simulink subsystem "ProcNav"  (R2020a)
settings: Solver=VariableStepAuto  StartTime=0.0  StopTime=10.0  RelTol=1e-3
undefined symbols (not defined in the file): DiscIntNeverNeededParam
libraries: aerolibutil x3, sharedtransform x2
settings Model: Creator=Lamarre  LastModifiedBy=lamarre

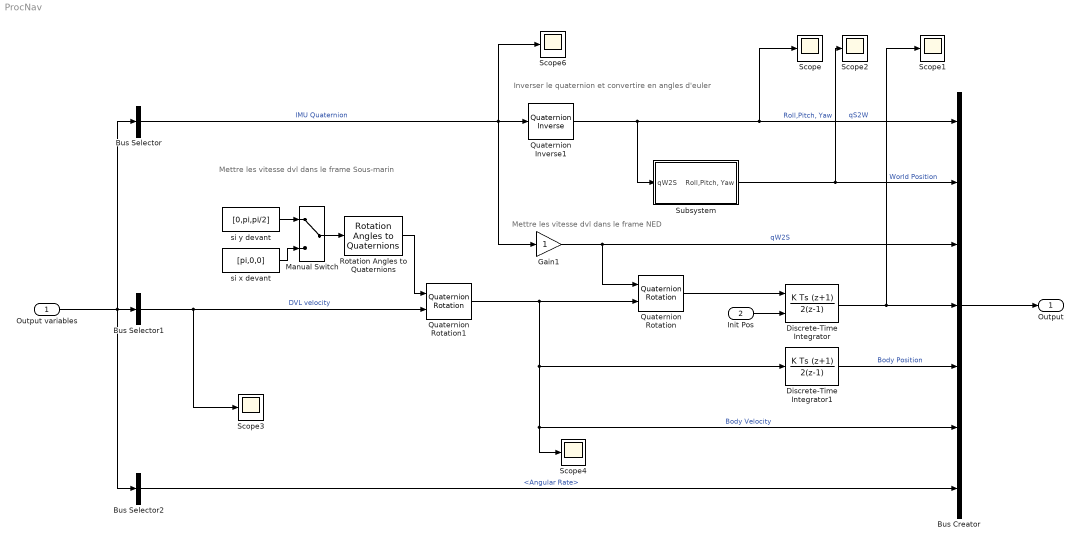
== system ProcNav ==
  note: Inverser le quaternion et convertire en angles d'euler
  note: Mettre les vitesse dvl dans le frame NED
  note: Mettre les vitesse dvl dans le frame Sous-marin
  Output variables : Inport
  Init Pos : Inport  Port=2
  Bus Creator : BusCreator  Inputs=7
  Bus Selector : BusSelector  OutputSignals=Quaternion  OutputAsBus=on
  Bus Selector1 : BusSelector  OutputSignals=DVL Velocity  OutputAsBus=on
  Bus Selector2 : BusSelector  OutputSignals=Angular Rate
  Discrete-Time Integrator : DiscreteIntegrator  IntegratorMethod=Integration: Trapezoidal  InitialConditionSource=external  SampleTime=-1  ICPrevOutput=DiscIntNeverNeededParam  ICPrevScaledInput=DiscIntNeverNeededParam
  Discrete-Time Integrator1 : DiscreteIntegrator  IntegratorMethod=Integration: Trapezoidal  SampleTime=-1  ICPrevOutput=DiscIntNeverNeededParam  ICPrevScaledInput=DiscIntNeverNeededParam
  Gain1 : Gain
  Manual Switch : ManualSwitch
  Quaternion Inverse1 : aerolibutil/Quaternion Inverse
  Quaternion Rotation : aerolibutil/Quaternion Rotation
  Quaternion Rotation1 : aerolibutil/Quaternion Rotation
  Rotation Angles to Quaternions : sharedtransform/Rotation Angles to Quaternions  rotationOrder=XYZ  aMode=aMode
      settings: SourceProductBaseCode=AE,PW,MT,VE,VP
  Scope{,1..4,6} (6 alike) : Scope
  Subsystem : Subsystem
  si x devant : Constant  Value=[pi,0,0]
  si y devant : Constant  Value=[0,pi,pi/2]
  Output : Outport
  wires:
  Bus Selector2/1 -> Bus Creator/7  "<Angular Rate>"
  Output variables/1 -> Bus Selector1/1, Bus Selector2/1, Bus Selector/1
  Bus Selector/1 -> Quaternion Inverse1/1, Gain1/1, Scope6/1  "IMU Quaternion"
  Discrete-Time Integrator1/1 -> Bus Creator/5  "Body Position"
  Discrete-Time Integrator/1 -> Bus Creator/4, Scope1/1  "World Position"
  Bus Creator/1 -> Output/1
  Quaternion Rotation/1 -> Discrete-Time Integrator/1
  Subsystem/1("Roll,Pitch, Yaw") -> Bus Creator/2, Scope2/1  "Roll,Pitch, Yaw"
  Quaternion Inverse1/1 -> Bus Creator/1, Scope/1, Subsystem/1(qW2S)  "qS2W"
  Gain1/1 -> Quaternion Rotation/1, Bus Creator/3  "qW2S"
  Init Pos/1 -> Discrete-Time Integrator/2
  Quaternion Rotation1/1 -> Quaternion Rotation/2, Discrete-Time Integrator1/1, Bus Creator/6, Scope4/1  "Body Velocity"
  Bus Selector1/1 -> Scope3/1, Quaternion Rotation1/2  "DVL velocity"
  Manual Switch/1 -> Rotation Angles to Quaternions/1
  si y devant/1 -> Manual Switch/1
  si x devant/1 -> Manual Switch/2
  Rotation Angles to Quaternions/1 -> Quaternion Rotation1/1

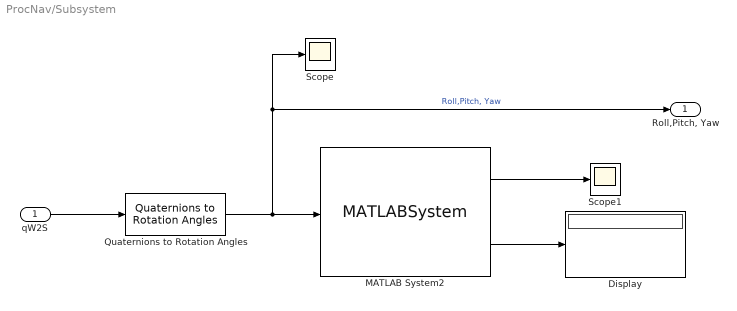
== system ProcNav/Subsystem ==
  qW2S : Inport
  Display : Display
  MATLAB System2 : MATLABSystem  System=DiscontinuityCheck  SimulateUsing=Code generation
      mask Type: DiscontinuityCheck
      mask Display:
      | disp('DiscontinuityCheck');
      | port_label('input',1,'angle');
      | port_label('output',1,'checkedAngle');
      | port_label('output',2,'tour');
  Quaternions to Rotation Angles : sharedtransform/Quaternions to Rotation Angles  rotationOrder=XYZ  aMode=aMode
      settings: SourceProductBaseCode=AE,PW,MT,VE,VP
  Scope : Scope
  Scope1 : Scope
  "Roll,Pitch, Yaw" : Outport
  wires:
  MATLAB System2/1 -> Scope1/1
  MATLAB System2/2 -> Display/1
  Quaternions to Rotation Angles/1 -> MATLAB System2/1, "Roll,Pitch, Yaw"/1, Scope/1  "Roll,Pitch, Yaw"
  qW2S/1 -> Quaternions to Rotation Angles/1
